simulink model "Final_Simulink_Model_assignment_2_PinA0_PinA1"  (R2022b)
settings: Solver=FixedStepAuto  StartTime=0.0  StopTime=inf  FixedStep=1e-3  RelTol=1e-3  EnableMultiTasking=on
undefined symbols (not defined in the file): A0, A1, ATR_PULSE_WIDTH, ATR_PUSLE_WIDTH, D0, D1, D10, D11, D12, D13, D2, D3, D4, D5, D6, D7, D8, D9, LRL, magnitude, PTA0, PTA1, PTA2, PTB2, PTB23, PTB3, PTB9, PTC16, PTC17, PTC2, PTC3, PTC4, PTD0, PTD1, PTD2, PTD3, REF_PERIOD, REF_PREIOD, VENT_PULSE_WIDTH
libraries: frdmk64flib x30, etargetslib x2, dspstat3 x1
(part 2 of 2)

== stateflow chart Final_Simulink_Model_assignment_2_PinA0_PinA1/Requirements Table1 ==
  (default) -> (junction 1073744884)
  (junction 1073744884) -> (junction 1073744885) : {
      | % SF_REQ_REV_07
      | }
  (junction 1073744885) -> (junction 1073744887) : {
      | % HEADER_ASSIGNMENTS
      |
      | }
  (junction 1073744887) -> (junction 1073744889) : {
      | % START_A_4
      | }
  (junction 1073744889) -> (junction 1073744891) : {
      | }
  (junction 1073744891) -> (junction 1073744893)
  (junction 1073744893) -> (junction 1073744895) : {
      | }
  (junction 1073744895) -> (junction 1073744897) : {
      | % END_A_4
      | }
  (junction 1073744897) -> (junction 1073744899) : {
      | % START_R_1
      | }
  (junction 1073744899) -> (junction 1073744901) : {
      | }
  (junction 1073744901) -> (junction 1073744903)
  (junction 1073744903) -> (junction 1073744905) [order 1] : [(((Mode) == (1)))]
  (junction 1073744903) -> (junction 1073744947) [order 2]
  (junction 1073744905) -> (junction 1073744907) : {
      |
      |
      | }
  (junction 1073744907) -> (junction 1073744909) : {
      | }
  (junction 1073744909) -> (junction 1073744911) : {
      | % START_R_7
      | }
  (junction 1073744911) -> (junction 1073744913) : {
      | }
  (junction 1073744913) -> (junction 1073744915)
  (junction 1073744915) -> (junction 1073744917) [order 1] : [duration((((State) == (1)))) >= 60000/LRL - ATR_PULSE_WIDTH]
  (junction 1073744915) -> (junction 1073744923) [order 2]
  (junction 1073744917) -> (junction 1073744919) : {
      | reqtable_postcondition((((ATR_PACE_CTRL) == (1))) && (((ATR_GND_CTRL) == (0))) && (((PACE_CHARGE_CTRL) == (0))) && (((PACE_GND_CTRL) == (1))), 'R:1.1');
      |
      |
      | }
  (junction 1073744919) -> (junction 1073744921) : {
      | }
  (junction 1073744921) -> (junction 1073744923)
  (junction 1073744923) -> (junction 1073744925)
  (junction 1073744925) -> (junction 1073744927) : {
      | % END_R_7
      | }
  (junction 1073744927) -> (junction 1073744929) : {
      | % START_R_10
      | }
  (junction 1073744929) -> (junction 1073744931) : {
      | }
  (junction 1073744931) -> (junction 1073744933)
  (junction 1073744933) -> (junction 1073744935) [order 1] : [duration((((State) == (2)))) >= ATR_PULSE_WIDTH]
  (junction 1073744933) -> (junction 1073744941) [order 2]
  (junction 1073744935) -> (junction 1073744937) : {
      | reqtable_postcondition((((ATR_PACE_CTRL) == (0))) && (((ATR_GND_CTRL) == (1))) && (((PACE_CHARGE_CTRL) == (1))) && (((PACE_GND_CTRL) == (1))), 'R:1.2');
      |
      |
      | }
  (junction 1073744937) -> (junction 1073744939) : {
      | }
  (junction 1073744939) -> (junction 1073744941)
  (junction 1073744941) -> (junction 1073744943)
  (junction 1073744943) -> (junction 1073744945) : {
      | % END_R_10
      | }
  (junction 1073744945) -> (junction 1073744947)
  (junction 1073744947) -> (junction 1073744949)
  (junction 1073744949) -> (junction 1073744951) : {
      | % END_R_1
      | }
  (junction 1073744951) -> (junction 1073744953) : {
      | % START_R_13
      | }
  (junction 1073744953) -> (junction 1073744955) : {
      | }
  (junction 1073744955) -> (junction 1073744957)
  (junction 1073744957) -> (junction 1073744959) [order 1] : [(((Mode) == (2)))]
  (junction 1073744957) -> (junction 1073745001) [order 2]
  (junction 1073744959) -> (junction 1073744961) : {
      |
      |
      | }
  (junction 1073744961) -> (junction 1073744963) : {
      | }
  (junction 1073744963) -> (junction 1073744965) : {
      | % START_R_16
      | }
  (junction 1073744965) -> (junction 1073744967) : {
      | }
  (junction 1073744967) -> (junction 1073744969)
  (junction 1073744969) -> (junction 1073744971) [order 1] : [duration((((State) == (1)))) >= 60000/LRL - VENT_PULSE_WIDTH]
  (junction 1073744969) -> (junction 1073744977) [order 2]
  (junction 1073744971) -> (junction 1073744973) : {
      | reqtable_postcondition((((PACE_CHARGE_CTRL) == (0))) && (((PACE_GND_CTRL) == (1))) && (((VENT_PACE_CTRL) == (1))) && (((VENT_GND_CTRL) == (0))), 'R:2.1');
      |
      |
      | }
  (junction 1073744973) -> (junction 1073744975) : {
      | }
  (junction 1073744975) -> (junction 1073744977)
  (junction 1073744977) -> (junction 1073744979)
  (junction 1073744979) -> (junction 1073744981) : {
      | % END_R_16
      | }
  (junction 1073744981) -> (junction 1073744983) : {
      | % START_R_19
      | }
  (junction 1073744983) -> (junction 1073744985) : {
      | }
  (junction 1073744985) -> (junction 1073744987)
  (junction 1073744987) -> (junction 1073744989) [order 1] : [duration((((State) == (2)))) >= VENT_PULSE_WIDTH]
  (junction 1073744987) -> (junction 1073744995) [order 2]
  (junction 1073744989) -> (junction 1073744991) : {
      | reqtable_postcondition((((PACE_CHARGE_CTRL) == (1))) && (((PACE_GND_CTRL) == (1))) && (((VENT_PACE_CTRL) == (0))) && (((VENT_GND_CTRL) == (1))), 'R:2.2');
      |
      |
      | }
  (junction 1073744991) -> (junction 1073744993) : {
      | }
  (junction 1073744993) -> (junction 1073744995)
  (junction 1073744995) -> (junction 1073744997)
  (junction 1073744997) -> (junction 1073744999) : {
      | % END_R_19
      | }
  (junction 1073744999) -> (junction 1073745001)
  (junction 1073745001) -> (junction 1073745003)
  (junction 1073745003) -> (junction 1073745005) : {
      | % END_R_13
      | }
  (junction 1073745005) -> (junction 1073745007) : {
      | % START_R_22
      | }
  (junction 1073745007) -> (junction 1073745009) : {
      | }
  (junction 1073745009) -> (junction 1073745011)
  (junction 1073745011) -> (junction 1073745013) [order 1] : [(((Mode) == (3)))]
  (junction 1073745011) -> (junction 1073745073) [order 2]
  (junction 1073745013) -> (junction 1073745015) : {
      |
      |
      | }
  (junction 1073745015) -> (junction 1073745017) : {
      | }
  (junction 1073745017) -> (junction 1073745019) : {
      | % START_R_25
      | }
  (junction 1073745019) -> (junction 1073745021) : {
      | }
  (junction 1073745021) -> (junction 1073745023)
  (junction 1073745023) -> (junction 1073745025) [order 1] : [duration((((State) == (1)))) >= 60000/LRL - ATR_PULSE_WIDTH]
  (junction 1073745023) -> (junction 1073745031) [order 2]
  (junction 1073745025) -> (junction 1073745027) : {
      | reqtable_postcondition((((ATR_PACE_CTRL) == (0))) && (((ATR_GND_CTRL) == (1))) && (((PACE_CHARGE_CTRL) == (1))) && (((PACE_GND_CTRL) == (1))) && (((FRONTEND_CTRL) == (1))), 'R:3.1');
      |
      |
      | }
  (junction 1073745027) -> (junction 1073745029) : {
      | }
  (junction 1073745029) -> (junction 1073745031)
  (junction 1073745031) -> (junction 1073745033)
  (junction 1073745033) -> (junction 1073745035) : {
      | % END_R_25
      | }
  (junction 1073745035) -> (junction 1073745037) : {
      | % START_R_28
      | }
  (junction 1073745037) -> (junction 1073745039) : {
      | }
  (junction 1073745039) -> (junction 1073745041)
  (junction 1073745041) -> (junction 1073745043) [order 1] : [duration((((State) == (2))) && (((ATR_CMP_DETECT) == (0)))) >= ATR_PULSE_WIDTH]
  (junction 1073745041) -> (junction 1073745049) [order 2]
  (junction 1073745043) -> (junction 1073745045) : {
      | reqtable_postcondition((((ATR_PACE_CTRL) == (1))) && (((ATR_GND_CTRL) == (0))) && (((PACE_CHARGE_CTRL) == (0))) && (((PACE_GND_CTRL) == (1))), 'R:3.2');
      |
      |
      | }
  (junction 1073745045) -> (junction 1073745047) : {
      | }
  (junction 1073745047) -> (junction 1073745049)
  (junction 1073745049) -> (junction 1073745051)
  (junction 1073745051) -> (junction 1073745053) : {
      | % END_R_28
      | }
  (junction 1073745053) -> (junction 1073745055) : {
      | % START_R_31
      | }
  (junction 1073745055) -> (junction 1073745057) : {
      | }
  (junction 1073745057) -> (junction 1073745059)
  (junction 1073745059) -> (junction 1073745061) [order 1] : [duration((((State) == (3))) && (((ATR_CMP_DETECT) == (1)))) >= ARP]
  (junction 1073745059) -> (junction 1073745067) [order 2]
  (junction 1073745061) -> (junction 1073745063) : {
      | reqtable_postcondition((((ATR_PACE_CTRL) == (0))) && (((ATR_GND_CTRL) == (1))) && (((PACE_CHARGE_CTRL) == (0))) && (((PACE_GND_CTRL) == (1))) && (((FRONTEND_CTRL) == (0))), 'R:3.3');
      |
      |
      | }
  (junction 1073745063) -> (junction 1073745065) : {
      | }
  (junction 1073745065) -> (junction 1073745067)
  (junction 1073745067) -> (junction 1073745069)
  (junction 1073745069) -> (junction 1073745071) : {
      | % END_R_31
      | }
  (junction 1073745071) -> (junction 1073745073)
  (junction 1073745073) -> (junction 1073745075)
  (junction 1073745075) -> (junction 1073745077) : {
      | % END_R_22
      | }
  (junction 1073745077) -> (junction 1073745079) : {
      | % START_R_34
      | }
  (junction 1073745079) -> (junction 1073745081) : {
      | }
  (junction 1073745081) -> (junction 1073745083)
  (junction 1073745083) -> (junction 1073745085) [order 1] : [(((Mode) == (4)))]
  (junction 1073745083) -> (junction 1073745145) [order 2]
  (junction 1073745085) -> (junction 1073745087) : {
      |
      |
      | }
  (junction 1073745087) -> (junction 1073745089) : {
      | }
  (junction 1073745089) -> (junction 1073745091) : {
      | % START_R_37
      | }
  (junction 1073745091) -> (junction 1073745093) : {
      | }
  (junction 1073745093) -> (junction 1073745095)
  (junction 1073745095) -> (junction 1073745097) [order 1] : [duration((((State) == (1)))) >= 60000/LRL - VENT_PULSE_WIDTH]
  (junction 1073745095) -> (junction 1073745103) [order 2]
  (junction 1073745097) -> (junction 1073745099) : {
      | reqtable_postcondition((((PACE_CHARGE_CTRL) == (1))) && (((PACE_GND_CTRL) == (1))) && (((VENT_PACE_CTRL) == (0))) && (((VENT_GND_CTRL) == (1))) && (((FRONTEND_CTRL) == (1))), 'R:4.1');
      |
      |
      | }
  (junction 1073745099) -> (junction 1073745101) : {
      | }
  (junction 1073745101) -> (junction 1073745103)
  (junction 1073745103) -> (junction 1073745105)
  (junction 1073745105) -> (junction 1073745107) : {
      | % END_R_37
      | }
  (junction 1073745107) -> (junction 1073745109) : {
      | % START_R_40
      | }
  (junction 1073745109) -> (junction 1073745111) : {
      | }
  (junction 1073745111) -> (junction 1073745113)
  (junction 1073745113) -> (junction 1073745115) [order 1] : [duration((((State) == (2))) && (((VENT_CMP_DETECT) == (0)))) >= VENT_PULSE_WIDTH]
  (junction 1073745113) -> (junction 1073745121) [order 2]
  (junction 1073745115) -> (junction 1073745117) : {
      | reqtable_postcondition((((PACE_CHARGE_CTRL) == (0))) && (((PACE_GND_CTRL) == (1))) && (((VENT_PACE_CTRL) == (1))) && (((VENT_GND_CTRL) == (0))), 'R:4.2');
      |
      |
      | }
  (junction 1073745117) -> (junction 1073745119) : {
      | }
  (junction 1073745119) -> (junction 1073745121)
  (junction 1073745121) -> (junction 1073745123)
  (junction 1073745123) -> (junction 1073745125) : {
      | % END_R_40
      | }
  (junction 1073745125) -> (junction 1073745127) : {
      | % START_R_43
      | }
  (junction 1073745127) -> (junction 1073745129) : {
      | }
  (junction 1073745129) -> (junction 1073745131)
  (junction 1073745131) -> (junction 1073745133) [order 1] : [duration((((State) == (3))) && (((VENT_CMP_DETECT) == (1)))) >= ARP]
  (junction 1073745131) -> (junction 1073745139) [order 2]
  (junction 1073745133) -> (junction 1073745135) : {
      | reqtable_postcondition((((PACE_CHARGE_CTRL) == (0))) && (((PACE_GND_CTRL) == (1))) && (((VENT_PACE_CTRL) == (0))) && (((VENT_GND_CTRL) == (1))) && (((FRONTEND_CTRL) == (0))), 'R:4.3');
      |
      |
      | }
  (junction 1073745135) -> (junction 1073745137) : {
      | }
  (junction 1073745137) -> (junction 1073745139)
  (junction 1073745139) -> (junction 1073745141)
  (junction 1073745141) -> (junction 1073745143) : {
      | % END_R_43
      | }
  (junction 1073745143) -> (junction 1073745145)
  (junction 1073745145) -> (junction 1073745147)
  (junction 1073745147) -> (junction 1073745149) : {
      | % END_R_34
      | }
  (junction 1073745149) -> (junction 1073745151) : {
      | % START_R_46
      | }
  (junction 1073745151) -> (junction 1073745153) : {
      | }
  (junction 1073745153) -> (junction 1073745155)
  (junction 1073745155) -> (junction 1073745157) [order 1] : [(((Mode) == (5)))]
  (junction 1073745155) -> (junction 1073745199) [order 2]
  (junction 1073745157) -> (junction 1073745159) : {
      |
      |
      | }
  (junction 1073745159) -> (junction 1073745161) : {
      | }
  (junction 1073745161) -> (junction 1073745163) : {
      | % START_R_49
      | }
  (junction 1073745163) -> (junction 1073745165) : {
      | }
  (junction 1073745165) -> (junction 1073745167)
  (junction 1073745167) -> (junction 1073745169) [order 1] : [duration((((State) == (1)))) >= 60000/Rate-ATR_PULSE_WIDTH]
  (junction 1073745167) -> (junction 1073745175) [order 2]
  (junction 1073745169) -> (junction 1073745171) : {
      | reqtable_postcondition((((ATR_PACE_CTRL) == (1))) && (((ATR_GND_CTRL) == (0))) && (((PACE_CHARGE_CTRL) == (0))) && (((PACE_GND_CTRL) == (1))), 'R:5.1');
      |
      |
      | }
  (junction 1073745171) -> (junction 1073745173) : {
      | }
  (junction 1073745173) -> (junction 1073745175)
  (junction 1073745175) -> (junction 1073745177)
  (junction 1073745177) -> (junction 1073745179) : {
      | % END_R_49
      | }
  (junction 1073745179) -> (junction 1073745181) : {
      | % START_R_52
      | }
  (junction 1073745181) -> (junction 1073745183) : {
      | }
  (junction 1073745183) -> (junction 1073745185)
  (junction 1073745185) -> (junction 1073745187) [order 1] : [duration((((State) == (2)))) >= ATR_PULSE_WIDTH]
  (junction 1073745185) -> (junction 1073745193) [order 2]
  (junction 1073745187) -> (junction 1073745189) : {
      | reqtable_postcondition((((ATR_PACE_CTRL) == (0))) && (((ATR_GND_CTRL) == (1))) && (((PACE_CHARGE_CTRL) == (1))) && (((PACE_GND_CTRL) == (1))), 'R:5.2');
      |
      |
      | }
  (junction 1073745189) -> (junction 1073745191) : {
      | }
  (junction 1073745191) -> (junction 1073745193)
  (junction 1073745193) -> (junction 1073745195)
  (junction 1073745195) -> (junction 1073745197) : {
      | % END_R_52
      | }
  (junction 1073745197) -> (junction 1073745199)
  (junction 1073745199) -> (junction 1073745201)
  (junction 1073745201) -> (junction 1073745203) : {
      | % END_R_46
      | }
  (junction 1073745203) -> (junction 1073745205) : {
      | % START_R_55
      | }
  (junction 1073745205) -> (junction 1073745207) : {
      | }
  (junction 1073745207) -> (junction 1073745209)
  (junction 1073745209) -> (junction 1073745211) [order 1] : [(((Mode) == (6)))]
  (junction 1073745209) -> (junction 1073745253) [order 2]
  (junction 1073745211) -> (junction 1073745213) : {
      |
      |
      | }
  (junction 1073745213) -> (junction 1073745215) : {
      | }
  (junction 1073745215) -> (junction 1073745217) : {
      | % START_R_58
      | }
  (junction 1073745217) -> (junction 1073745219) : {
      | }
  (junction 1073745219) -> (junction 1073745221)
  (junction 1073745221) -> (junction 1073745223) [order 1] : [duration((((State) == (1)))) >= 60000/ Rate- VENT_PULSE_WIDTH]
  (junction 1073745221) -> (junction 1073745229) [order 2]
  (junction 1073745223) -> (junction 1073745225) : {
      | reqtable_postcondition((((PACE_CHARGE_CTRL) == (0))) && (((PACE_GND_CTRL) == (1))) && (((VENT_PACE_CTRL) == (1))) && (((VENT_GND_CTRL) == (0))), 'R:6.1');
      |
      |
      | }
  (junction 1073745225) -> (junction 1073745227) : {
      | }
  (junction 1073745227) -> (junction 1073745229)
  (junction 1073745229) -> (junction 1073745231)
  (junction 1073745231) -> (junction 1073745233) : {
      | % END_R_58
      | }
  (junction 1073745233) -> (junction 1073745235) : {
      | % START_R_61
      | }
  (junction 1073745235) -> (junction 1073745237) : {
      | }
  (junction 1073745237) -> (junction 1073745239)
  (junction 1073745239) -> (junction 1073745241) [order 1] : [duration((((State) == (2)))) >= VENT_PULSE_WIDTH]
  (junction 1073745239) -> (junction 1073745247) [order 2]
  (junction 1073745241) -> (junction 1073745243) : {
      | reqtable_postcondition((((PACE_CHARGE_CTRL) == (1))) && (((PACE_GND_CTRL) == (1))) && (((VENT_PACE_CTRL) == (0))) && (((VENT_GND_CTRL) == (1))), 'R:6.2');
      |
      |
      | }
  (junction 1073745243) -> (junction 1073745245) : {
      | }
  (junction 1073745245) -> (junction 1073745247)
  (junction 1073745247) -> (junction 1073745249)
  (junction 1073745249) -> (junction 1073745251) : {
      | % END_R_61
      | }
  (junction 1073745251) -> (junction 1073745253)
  (junction 1073745253) -> (junction 1073745255)
  (junction 1073745255) -> (junction 1073745257) : {
      | % END_R_55
      | }
  (junction 1073745257) -> (junction 1073745259) : {
      | % START_R_64
      | }
  (junction 1073745259) -> (junction 1073745261) : {
      | }
  (junction 1073745261) -> (junction 1073745263)
  (junction 1073745263) -> (junction 1073745265) [order 1] : [(((Mode) == (7)))]
  (junction 1073745263) -> (junction 1073745325) [order 2]
  (junction 1073745265) -> (junction 1073745267) : {
      |
      |
      | }
  (junction 1073745267) -> (junction 1073745269) : {
      | }
  (junction 1073745269) -> (junction 1073745271) : {
      | % START_R_67
      | }
  (junction 1073745271) -> (junction 1073745273) : {
      | }
  (junction 1073745273) -> (junction 1073745275)
  (junction 1073745275) -> (junction 1073745277) [order 1] : [duration((((State) == (1)))) >= 60000/Rate-ATR_PULSE_WIDTH-ARP]
  (junction 1073745275) -> (junction 1073745283) [order 2]
  (junction 1073745277) -> (junction 1073745279) : {
      | reqtable_postcondition((((ATR_PACE_CTRL) == (0))) && (((ATR_GND_CTRL) == (1))) && (((PACE_CHARGE_CTRL) == (1))) && (((PACE_GND_CTRL) == (1))) && (((FRONTEND_CTRL) == (1))), 'R:7.1');
      |
      |
      | }
  (junction 1073745279) -> (junction 1073745281) : {
      | }
  (junction 1073745281) -> (junction 1073745283)
  (junction 1073745283) -> (junction 1073745285)
  (junction 1073745285) -> (junction 1073745287) : {
      | % END_R_67
      | }
  (junction 1073745287) -> (junction 1073745289) : {
      | % START_R_70
      | }
  (junction 1073745289) -> (junction 1073745291) : {
      | }
  (junction 1073745291) -> (junction 1073745293)
  (junction 1073745293) -> (junction 1073745295) [order 1] : [duration((((State) == (2))) && (((ATR_CMP_DETECT) == (0)))) >= ARP]
  (junction 1073745293) -> (junction 1073745301) [order 2]
  (junction 1073745295) -> (junction 1073745297) : {
      | reqtable_postcondition((((ATR_PACE_CTRL) == (1))) && (((ATR_GND_CTRL) == (0))) && (((PACE_CHARGE_CTRL) == (0))) && (((PACE_GND_CTRL) == (1))), 'R:7.2');
      |
      |
      | }
  (junction 1073745297) -> (junction 1073745299) : {
      | }
  (junction 1073745299) -> (junction 1073745301)
  (junction 1073745301) -> (junction 1073745303)
  (junction 1073745303) -> (junction 1073745305) : {
      | % END_R_70
      | }
  (junction 1073745305) -> (junction 1073745307) : {
      | % START_R_73
      | }
  (junction 1073745307) -> (junction 1073745309) : {
      | }
  (junction 1073745309) -> (junction 1073745311)
  (junction 1073745311) -> (junction 1073745313) [order 1] : [duration((((State) == (3))) && (((ATR_CMP_DETECT) == (1)))) >= ARP]
  (junction 1073745311) -> (junction 1073745319) [order 2]
  (junction 1073745313) -> (junction 1073745315) : {
      | reqtable_postcondition((((ATR_PACE_CTRL) == (0))) && (((ATR_GND_CTRL) == (1))) && (((PACE_CHARGE_CTRL) == (0))) && (((PACE_GND_CTRL) == (1))) && (((FRONTEND_CTRL) == (0))), 'R:7.3');
      |
      |
      | }
  (junction 1073745315) -> (junction 1073745317) : {
      | }
  (junction 1073745317) -> (junction 1073745319)
  (junction 1073745319) -> (junction 1073745321)
  (junction 1073745321) -> (junction 1073745323) : {
      | % END_R_73
      | }
  (junction 1073745323) -> (junction 1073745325)
  (junction 1073745325) -> (junction 1073745327)
  (junction 1073745327) -> (junction 1073745329) : {
      | % END_R_64
      | }
  (junction 1073745329) -> (junction 1073745331) : {
      | % START_R_76
      | }
  (junction 1073745331) -> (junction 1073745333) : {
      | }
  (junction 1073745333) -> (junction 1073745335)
  (junction 1073745335) -> (junction 1073745337) [order 1] : [(((Mode) == (8)))]
  (junction 1073745335) -> (junction 1073745397) [order 2]
  (junction 1073745337) -> (junction 1073745339) : {
      |
      |
      | }
  (junction 1073745339) -> (junction 1073745341) : {
      | }
  (junction 1073745341) -> (junction 1073745343) : {
      | % START_R_79
      | }
  (junction 1073745343) -> (junction 1073745345) : {
      | }
  (junction 1073745345) -> (junction 1073745347)
  (junction 1073745347) -> (junction 1073745349) [order 1] : [duration((((State) == (1)))) >= 60000/Rate-VENT_PULSE_WIDTH-VRP]
  (junction 1073745347) -> (junction 1073745355) [order 2]
  (junction 1073745349) -> (junction 1073745351) : {
      | reqtable_postcondition((((PACE_CHARGE_CTRL) == (1))) && (((PACE_GND_CTRL) == (1))) && (((VENT_PACE_CTRL) == (0))) && (((VENT_GND_CTRL) == (1))) && (((FRONTEND_CTRL) == (1))), 'R:8.1');
      |
      |
      | }
  (junction 1073745351) -> (junction 1073745353) : {
      | }
  (junction 1073745353) -> (junction 1073745355)
  (junction 1073745355) -> (junction 1073745357)
  (junction 1073745357) -> (junction 1073745359) : {
      | % END_R_79
      | }
  (junction 1073745359) -> (junction 1073745361) : {
      | % START_R_85
      | }
  (junction 1073745361) -> (junction 1073745363) : {
      | }
  (junction 1073745363) -> (junction 1073745365)
  (junction 1073745365) -> (junction 1073745367) [order 1] : [duration((((State) == (2))) && (((VENT_CMP_DETECT) == (0)))) >= VRP]
  (junction 1073745365) -> (junction 1073745373) [order 2]
  (junction 1073745367) -> (junction 1073745369) : {
      | reqtable_postcondition((((PACE_CHARGE_CTRL) == (0))) && (((PACE_GND_CTRL) == (1))) && (((VENT_PACE_CTRL) == (1))) && (((VENT_GND_CTRL) == (0))), 'R:8.2');
      |
      |
      | }
  (junction 1073745369) -> (junction 1073745371) : {
      | }
  (junction 1073745371) -> (junction 1073745373)
  (junction 1073745373) -> (junction 1073745375)
  (junction 1073745375) -> (junction 1073745377) : {
      | % END_R_85
      | }
  (junction 1073745377) -> (junction 1073745379) : {
      | % START_R_88
      | }
  (junction 1073745379) -> (junction 1073745381) : {
      | }
  (junction 1073745381) -> (junction 1073745383)
  (junction 1073745383) -> (junction 1073745385) [order 1] : [duration((((State) == (3))) && (((VENT_CMP_DETECT) == (1)))) >= VRP]
  (junction 1073745383) -> (junction 1073745391) [order 2]
  (junction 1073745385) -> (junction 1073745387) : {
      | reqtable_postcondition((((PACE_CHARGE_CTRL) == (0))) && (((PACE_GND_CTRL) == (1))) && (((VENT_GND_CTRL) == (1))) && (((FRONTEND_CTRL) == (0))), 'R:8.3');
      |
      |
      | }
  (junction 1073745387) -> (junction 1073745389) : {
      | }
  (junction 1073745389) -> (junction 1073745391)
  (junction 1073745391) -> (junction 1073745393)
  (junction 1073745393) -> (junction 1073745395) : {
      | % END_R_88
      | }
  (junction 1073745395) -> (junction 1073745397)
  (junction 1073745397) -> (junction 1073745399)
  (junction 1073745399) -> (junction 1073745401) : {
      | % END_R_76
      | }
  data: State input; FRONTEND_CTRL input; VENT_PACE_CTRL input; VENT_GND_CTRL input; ATR_PACE_CTRL input; ATR_GND_CTRL input; PACE_CHARGE_CTRL input; PACE_GND_CTRL input; Mode input double; ATR_CMP_DETECT input; VENT_CMP_DETECT input; ARP constant double; VRP constant double; Rate constant double; LRL constant double; VENT_PULSE_WIDTH constant double; ATR_PULSE_WIDTH constant double
